simulink model "Pad_Disc_model (1)"  (R2023a)
settings: Solver=VariableStepAuto  StartTime=0.0  StopTime=0.5  RelTol=1e-3
libraries: simulink_extras x3

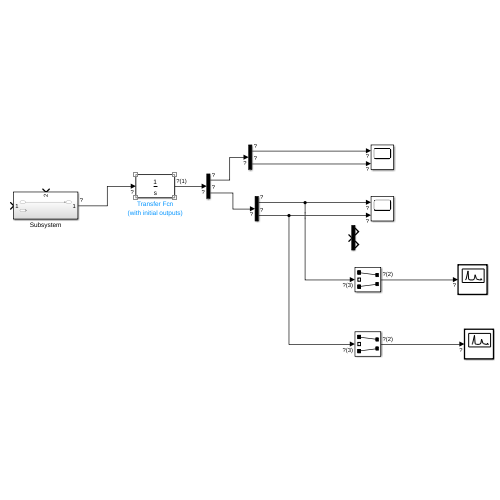
[thumbnail: Simulink's stored preview of the top-level diagram]
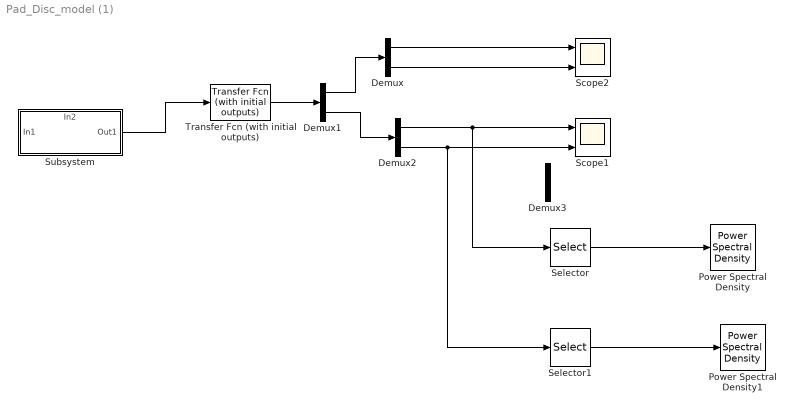
== system Pad_Disc_model (1) ==
  Demux{,1..3} (4 alike) : Demux  Outputs=2
  Power Spectral Density : simulink_extras/Additional Sinks/Power Spectral Density  npts=128  fftpts=512  HowOften=64  sampleT=0.1
  Power Spectral Density1 : simulink_extras/Additional Sinks/Power Spectral Density  npts=128  fftpts=512  HowOften=64  sampleT=0.1
  Scope1 : Scope  NumInputPorts=2
  Scope2 : Scope  NumInputPorts=2
  Selector : Selector  InputPortWidth=3  IndexOptions=Index vector (dialog)  Indices=[1 3]  OutputSizes=1
  Selector1 : Selector  InputPortWidth=3  IndexOptions=Index vector (dialog)  Indices=[1 3]  OutputSizes=1
  Subsystem : Subsystem
      settings: PortSchema="{\"entries\":[{\"content\":{\"sides\":[{\"content\":{\"connectorIds\":[\"In1\"]},\"type\":\"ConnectorPlacement.EquallySpacedRectSide\",\"uuid\":\"9acc9ba7-d7f5-4e53-815c-41beb3887c21\"},{\"content\":{\"connectorIds\":[\"Out1\"],\"side\":\"RIGHT\"},\"type\":\"ConnectorPlacement.EquallySpacedRectSide\",\"uuid\":\"6d57aca9-9a99-48c6-822b-4217dfd49061\"},{\"content\":{\"connectorIds\":[\"In2\"],\"side\":\"TOP\"},\"type\":\"ConnectorPlacement.EquallySpacedRectSide\",\"uuid\":\"6e551340-043b-4dde-814e-9a70bdfaccbe\"}]},\"type\":\"ConnectorPlacement.EquallySpacedConnector\",\"uuid\":\"01d10ea9-cee1-4902-a86f-5e7ac495c067\"}],\"packageUris\":[\"http://schema.mathworks.com/mf0/Connector/R2020b\"],\"version\":\"1.0\"}"
  Transfer Fcn (with initial outputs) : simulink_extras/Additional Linear/Transfer Fcn (with initial outputs)  N=[1]  D="[1  0]"  Y0=0  U0=0
  wires:
  Subsystem/1(Out1) -> Transfer Fcn (with initial outputs)/1
  Transfer Fcn (with initial outputs)/1 -> Demux1/1
  Demux1/1 -> Demux/1
  Demux1/2 -> Demux2/1
  Demux/2 -> Scope2/2
  Demux2/1 -> Selector/1, Scope1/1
  Demux2/2 -> Selector1/1, Scope1/2
  Demux/1 -> Scope2/1
  Selector/1 -> Power Spectral Density/1
  Selector1/1 -> Power Spectral Density1/1

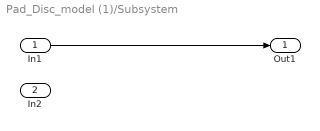
== system Pad_Disc_model (1)/Subsystem ==
  In1 : Inport
  In2 : Inport  Port=2
  Out1 : Outport
  wires:
  In1/1 -> Out1/1
